simulink model "output_feedback_gazebo"  (R2015b)
settings: Solver=ode3  StartTime=0.0  StopTime=inf  FixedStep=0.01  RelTol=1e-3
values from neighbouring files (symbols this model uses):
  Kx = KK(:,1:8)    [drone_config.m]
  Ky = KK(:,9:12)    [drone_config.m]
undefined symbols (not defined in the file or in its folder): W, X, Y, Z
libraries: simulink_extras x3, robotlib x3, aerolibtransform2 x1, simulink x1, aerolibanimutils x1
settings Model: Creator=rcasado  LastModifiedBy=rcasado
settings DataIOCC: SaveFormat=Array
settings DebuggingCC: MultiTaskRateTransMsg=warning
settings HardwareCC: ProdBitPerPointer=32  ProdLargestAtomicFloat=None  ProdIntDivRoundTo=Undefined  ProdEndianess=Unspecified  ProdWordSize=32  ProdHWDeviceType=32-bit Generic
settings GRTTargetCC: GeneratePreprocessorConditionals=Disable all
settings ConfigComp: CovModelRefEnable=Off

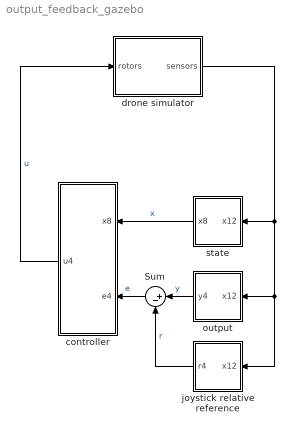
== system output_feedback_gazebo ==
  Sum : Sum  Inputs=|+-
  controller : Subsystem
  drone simulator : Subsystem
  joystick relative reference : Subsystem
  output : Subsystem
  state : Subsystem
  wires:
  drone simulator/1(sensors) -> joystick relative reference/1(x12), output/1(x12), state/1(x12)
  joystick relative reference/1(r4) -> Sum/2  "r"
  controller/1(u4) -> drone simulator/1(rotors)  "u"
  output/1(y4) -> Sum/1  "y"
  state/1(x8) -> controller/1(x8)  "x"
  Sum/1 -> controller/2(e4)  "e"

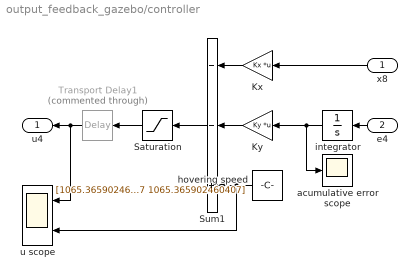
== system output_feedback_gazebo/controller ==
  x8 : Inport
  e4 : Inport  Port=2
  Kx : Gain  Gain=Kx  Multiplication=Matrix(K*u)
  Ky : Gain  Gain=Ky  Multiplication=Matrix(K*u)
  Saturation : Saturate  UpperLimit=1650  LowerLimit=0
  Sum1 : Sum  Inputs=--+
  Transport Delay1 : TransportDelay  Commented=through  DelayTime=0.05
  acumulative error scope : Scope
  hovering speed : Constant  Value=[1065.365902460407 1065.365902460407 1065.365902460407 1065.365902460407]
  integrator : Integrator
  u scope : Scope  NumInputPorts=2
  u4 : Outport
  wires:
  Saturation/1 -> Transport Delay1/1
  Kx/1 -> Sum1/1
  x8/1 -> Kx/1
  hovering speed/1 -> u scope/2, Sum1/3
  Sum1/1 -> Saturation/1
  Transport Delay1/1 -> u scope/1, u4/1
  e4/1 -> integrator/1
  Ky/1 -> Sum1/2
  integrator/1 -> Ky/1, acumulative error scope/1

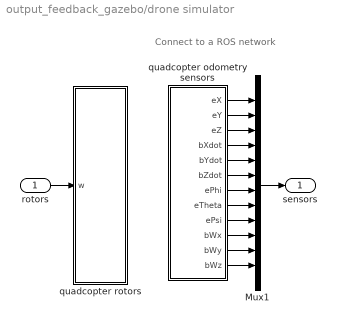
== system output_feedback_gazebo/drone simulator ==
  note: Connect to a
      | ROS network
  rotors : Inport
  Mux1 : Mux  Inputs=12
  quadcopter odometry sensors : Subsystem
  quadcopter rotors : Subsystem
  sensors : Outport
  wires:
  quadcopter odometry sensors/1(eX) -> Mux1/1
  rotors/1 -> quadcopter rotors/1(w)
  quadcopter odometry sensors/2(eY) -> Mux1/2
  quadcopter odometry sensors/3(eZ) -> Mux1/3
  Mux1/1 -> sensors/1
  quadcopter odometry sensors/4(bXdot) -> Mux1/4
  quadcopter odometry sensors/5(bYdot) -> Mux1/5
  quadcopter odometry sensors/6(bZdot) -> Mux1/6
  quadcopter odometry sensors/7(ePhi) -> Mux1/7
  quadcopter odometry sensors/8(eTheta) -> Mux1/8
  quadcopter odometry sensors/9(ePsi) -> Mux1/9
  quadcopter odometry sensors/10(bWx) -> Mux1/10
  quadcopter odometry sensors/11(bWy) -> Mux1/11
  quadcopter odometry sensors/12(bWz) -> Mux1/12

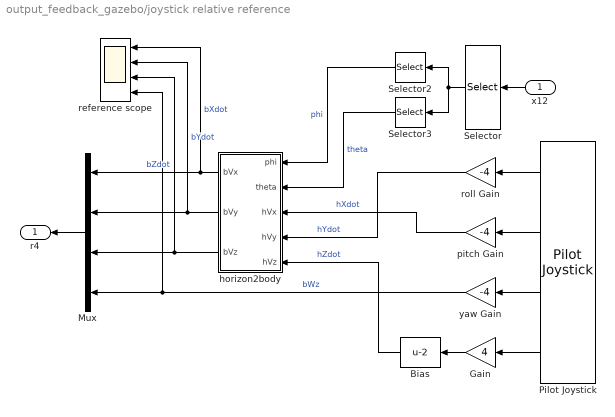
== system output_feedback_gazebo/joystick relative reference ==
  x12 : Inport
  Bias : Bias  Bias=-2
  Gain : Gain  Gain=4
  Mux : Mux
  Pilot Joystick : aerolibanimutils/Pilot Joystick  JoystickID=Joystick1  OutputConfiguration=FourAxis  SampleTime=0.1
  Selector : Selector  InputPortWidth=12  IndexOptions=Index vector (dialog)  Indices=[7,8]  OutputSizes=1
  Selector2 : Selector  InputPortWidth=2  IndexOptions=Index vector (dialog)  Indices=[1]  OutputSizes=1
  Selector3 : Selector  InputPortWidth=2  IndexOptions=Index vector (dialog)  Indices=[2]  OutputSizes=1
  horizon2body : Subsystem
  pitch Gain : Gain  Gain=-4
  reference scope : Scope  NumInputPorts=4
  roll Gain : Gain  Gain=-4
  yaw Gain : Gain  Gain=-4
  r4 : Outport
  wires:
  Mux/1 -> r4/1
  yaw Gain/1 -> reference scope/4, Mux/4  "bWz"
  pitch Gain/1 -> horizon2body/3(hVx)  "hXdot"
  Pilot Joystick/1 -> roll Gain/1
  Pilot Joystick/2 -> pitch Gain/1
  Pilot Joystick/3 -> yaw Gain/1
  Gain/1 -> Bias/1
  roll Gain/1 -> horizon2body/4(hVy)  "hYdot"
  Pilot Joystick/4 -> Gain/1
  Selector2/1 -> horizon2body/1(phi)  "phi"
  Selector3/1 -> horizon2body/2(theta)  "theta"
  x12/1 -> Selector/1
  Bias/1 -> horizon2body/5(hVz)  "hZdot"
  horizon2body/2(bVy) -> Mux/2, reference scope/2  "bYdot"
  horizon2body/1(bVx) -> Mux/1, reference scope/1  "bXdot"
  horizon2body/3(bVz) -> Mux/3, reference scope/3  "bZdot"
  Selector/1 -> Selector2/1, Selector3/1

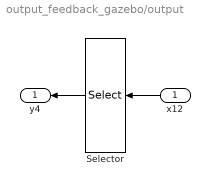
== system output_feedback_gazebo/output ==
  x12 : Inport
  Selector : Selector  InputPortWidth=12  IndexOptions=Index vector (dialog)  Indices=[4 5 6 12]  OutputSizes=1
  y4 : Outport
  wires:
  x12/1 -> Selector/1
  Selector/1 -> y4/1

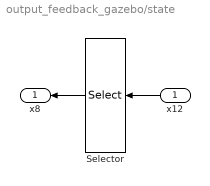
== system output_feedback_gazebo/state ==
  x12 : Inport
  Selector : Selector  InputPortWidth=12  IndexOptions=Index vector (dialog)  Indices=[7 8 10 11 12 4 5 6]  OutputSizes=1
  x8 : Outport
  wires:
  x12/1 -> Selector/1
  Selector/1 -> x8/1

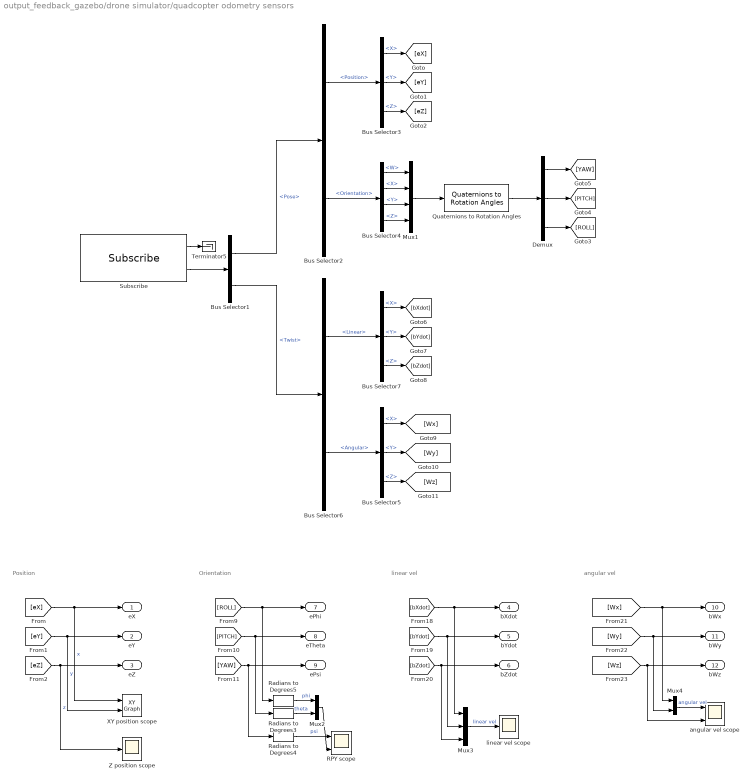
== system output_feedback_gazebo/drone simulator/quadcopter odometry sensors ==
  note: linear vel
  note: Position
  note: Orientation
  note: angular vel
  Bus Selector1 : BusSelector  DialogController=Simulink.DDGSource_BusSelector  OutputSignals=Pose,Twist
  Bus Selector2 : BusSelector  DialogController=Simulink.DDGSource_BusSelector  OutputSignals=Position,Orientation
  Bus Selector3 : BusSelector  DialogController=Simulink.DDGSource_BusSelector  OutputSignals=X,Y,Z
  Bus Selector4 : BusSelector  DialogController=Simulink.DDGSource_BusSelector  OutputSignals=W,X,Y,Z
  Bus Selector5 : BusSelector  DialogController=Simulink.DDGSource_BusSelector  OutputSignals=X,Y,Z
  Bus Selector6 : BusSelector  DialogController=Simulink.DDGSource_BusSelector  OutputSignals=Linear,Angular
  Bus Selector7 : BusSelector  DialogController=Simulink.DDGSource_BusSelector  OutputSignals=X,Y,Z
  Demux : Demux  Outputs=3
  Mux1 : Mux
  Mux2 : Mux  Inputs=2
  Mux3 : Mux  Inputs=3
  Mux4 : Mux  Inputs=2
  Quaternions to Rotation Angles : aerolibtransform2/Quaternions to Rotation Angles  rotationOrder=ZYX
  RPY scope : Scope  NumInputPorts=2
  Radians to Degrees3 : simulink_extras/Transformations/Radians to Degrees
  Radians to Degrees4 : simulink_extras/Transformations/Radians to Degrees
  Radians to Degrees5 : simulink_extras/Transformations/Radians to Degrees
  Subscribe : robotlib/Subscribe  SourceLibraryInfo=This block requires Robotics System Toolbox  topicSource=Specify your own  topic=/quadcopter/odometry  messageType=gazebo_msgs/ModelState  sampleTime=-1  messageQueueLength=51
  Terminator5 : Terminator
  XY position scope : simulink/Sinks/XY Graph  xmin=-10  xmax=10  ymin=-10  ymax=10  st=-1
  Z position scope : Scope
  angular vel scope : Scope  NumInputPorts=2
  linear vel scope : Scope
  eX : Outport
  eY : Outport  Port=2
  eZ : Outport  Port=3
  bXdot : Outport  Port=4
  bYdot : Outport  Port=5
  bZdot : Outport  Port=6
  ePhi : Outport  Port=7
  eTheta : Outport  Port=8
  ePsi : Outport  Port=9
  bWx : Outport  Port=10
  bWy : Outport  Port=11
  bWz : Outport  Port=12
  wires:
  Subscribe/2 -> Bus Selector1/1
  Bus Selector1/1 -> Bus Selector2/1  "<Pose>"
  Bus Selector1/2 -> Bus Selector6/1  "<Twist>"
  Subscribe/1 -> Terminator5/1
  Bus Selector2/1 -> Bus Selector3/1  "<Position>"
  Bus Selector3/1 -> [eX]  "<X>"
  Bus Selector3/2 -> [eY]  "<Y>"
  Bus Selector3/3 -> [eZ]  "<Z>"
  [eX] -> XY position scope/1, eX/1  "x"
  [eY] -> XY position scope/2, eY/1  "y"
  [eZ] -> Z position scope/1, eZ/1  "z"
  Bus Selector2/2 -> Bus Selector4/1  "<Orientation>"
  Quaternions to Rotation Angles/1 -> Demux/1
  [PITCH] -> eTheta/1, Radians to Degrees3/1
  [ROLL] -> ePhi/1, Radians to Degrees5/1
  Demux/1 -> [YAW]
  Demux/3 -> [ROLL]
  Demux/2 -> [PITCH]
  Mux1/1 -> Quaternions to Rotation Angles/1
  Bus Selector4/1 -> Mux1/1  "<W>"
  Bus Selector4/2 -> Mux1/2  "<X>"
  Bus Selector4/3 -> Mux1/3  "<Y>"
  Bus Selector4/4 -> Mux1/4  "<Z>"
  Bus Selector6/1 -> Bus Selector7/1  "<Linear>"
  Bus Selector7/1 -> [bXdot]  "<X>"
  Bus Selector7/2 -> [bYdot]  "<Y>"
  Bus Selector7/3 -> [bZdot]  "<Z>"
  Bus Selector6/2 -> Bus Selector5/1  "<Angular>"
  Bus Selector5/1 -> [Wx]  "<X>"
  Bus Selector5/2 -> [Wy]  "<Y>"
  Bus Selector5/3 -> [Wz]  "<Z>"
  Mux3/1 -> linear vel scope/1  "linear vel"
  Mux4/1 -> angular vel scope/1  "angular vel"
  [Wx] -> bWx/1, Mux4/1
  [Wy] -> bWy/1, Mux4/2
  [Wz] -> angular vel scope/2, bWz/1
  [bXdot] -> Mux3/1, bXdot/1
  [bYdot] -> Mux3/2, bYdot/1
  [bZdot] -> Mux3/3, bZdot/1
  [YAW] -> Radians to Degrees4/1, ePsi/1
  Radians to Degrees3/1 -> Mux2/2  "theta"
  Radians to Degrees4/1 -> RPY scope/1  "psi"
  Radians to Degrees5/1 -> Mux2/1  "phi"
  Mux2/1 -> RPY scope/2

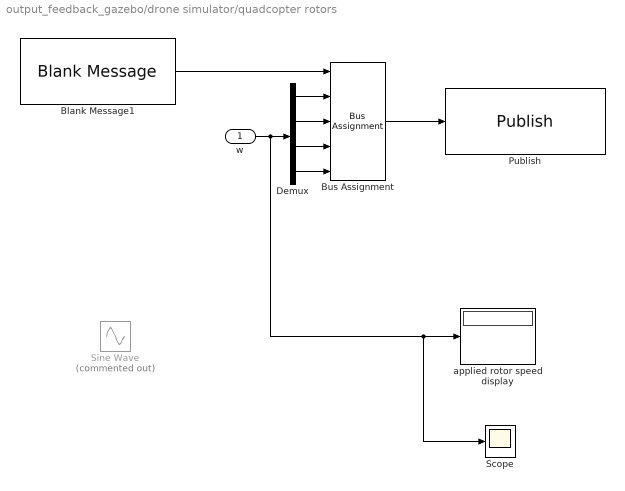
== system output_feedback_gazebo/drone simulator/quadcopter rotors ==
  w : Inport
  Blank Message1 : robotlib/Blank Message  SourceLibraryInfo=This block requires Robotics System Toolbox  messageType=geometry_msgs/Quaternion  SampleTime=0.01
  Bus Assignment : BusAssignment  AssignedSignals=X,Y,Z,W
  Demux : Demux
  Publish : robotlib/Publish  SourceLibraryInfo=This block requires Robotics System Toolbox  topicSource=Select from ROS network  topic=/quadcopter/rotor_speeds  messageType=geometry_msgs/Quaternion  messageQueueLength=105
  Scope : Scope
  Sine Wave : Sin  Commented=on  Amplitude=500  Bias=1000  Frequency=2*pi/10  Phase=-pi/2  SampleTime=0
  applied rotor speed display : Display
      settings: Decimation=5
  wires:
  Bus Assignment/1 -> Publish/1
  w/1 -> Scope/1, applied rotor speed display/1, Demux/1
  Blank Message1/1 -> Bus Assignment/1
  Demux/4 -> Bus Assignment/5
  Demux/3 -> Bus Assignment/4
  Demux/2 -> Bus Assignment/3
  Demux/1 -> Bus Assignment/2

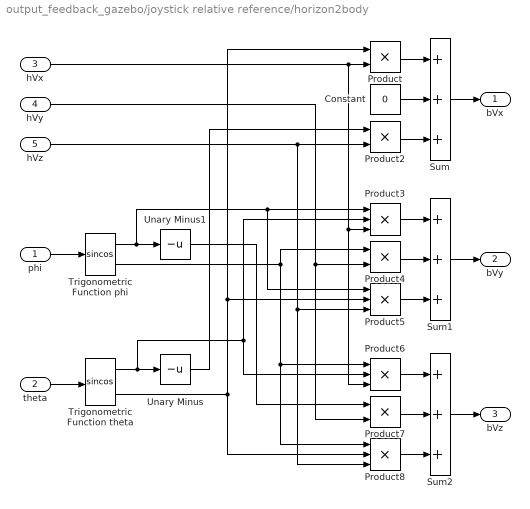
== system output_feedback_gazebo/joystick relative reference/horizon2body ==
  phi : Inport
  theta : Inport  Port=2
  hVx : Inport  Port=3
  hVy : Inport  Port=4
  hVz : Inport  Port=5
  Constant : Constant  Value=0
  Product{,2,4,7} (4 alike) : Product
  Product{3,5..6,8} (4 alike) : Product  Inputs=3
  Sum : Sum  Inputs=3
  Sum1 : Sum  Inputs=3
  Sum2 : Sum  Inputs=3
  Trigonometric Function phi : Trigonometry  Operator=sincos
  Trigonometric Function theta : Trigonometry  Operator=sincos
  Unary Minus : UnaryMinus
  Unary Minus1 : UnaryMinus
  bVx : Outport
  bVy : Outport  Port=2
  bVz : Outport  Port=3
  wires:
  theta/1 -> Trigonometric Function theta/1
  phi/1 -> Trigonometric Function phi/1
  Trigonometric Function phi/2 -> Product4/1, Product8/1, Product6/1
  Trigonometric Function theta/2 -> Product8/2, Product/1, Product5/2
  Trigonometric Function theta/1 -> Product3/2, Product6/2, Unary Minus/1
  Trigonometric Function phi/1 -> Unary Minus1/1, Product5/1, Product3/1
  Sum/1 -> bVx/1
  Sum1/1 -> bVy/1
  Sum2/1 -> bVz/1
  Product/1 -> Sum/1
  Constant/1 -> Sum/2
  Product2/1 -> Sum/3
  Product3/1 -> Sum1/1
  Product4/1 -> Sum1/2
  Product5/1 -> Sum1/3
  Product6/1 -> Sum2/1
  Product7/1 -> Sum2/2
  Product8/1 -> Sum2/3
  hVx/1 -> Product6/3, Product3/3, Product/2
  hVy/1 -> Product7/2, Product4/2
  hVz/1 -> Product8/3, Product5/3, Product2/2
  Unary Minus/1 -> Product2/1
  Unary Minus1/1 -> Product7/1
